simulink model "EDTetherSim"  (R2018b)
settings: Solver=VariableStepAuto  StartTime=0.0  StopTime=86400  RelTol=1e-3
settings Model: Creator=walte102  LastModifiedBy=walte102

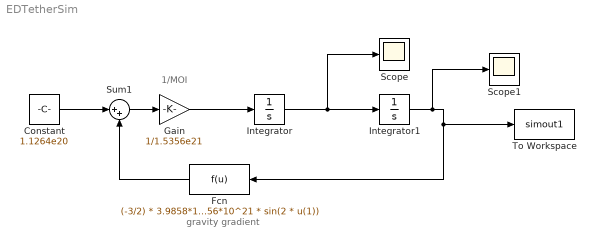
== system EDTetherSim ==
  note: 1/MOI
  note: gravity gradient
  Constant : Constant  Value=1.1264e20
  Fcn : Fcn  Expr=(-3/2) * 3.9858*10^14 / (7306 * 1000)^3 * 1.5356*10^21 * sin(2 * u(1))
  Gain : Gain  Gain=1/1.5356e21
  Integrator : Integrator
  Integrator1 : Integrator
  Scope : Scope
  Scope1 : Scope
  Sum1 : Sum  Inputs=|++
  To Workspace : ToWorkspace  VariableName=simout1  SaveFormat=Structure With Time  SampleTime=-1
  wires:
  Integrator/1 -> Scope/1, Integrator1/1
  Gain/1 -> Integrator/1
  Integrator1/1 -> Scope1/1, To Workspace/1, Fcn/1
  Sum1/1 -> Gain/1
  Constant/1 -> Sum1/1
  Fcn/1 -> Sum1/2
